simulink library "GEJenbacherJ620"  (Simulink 8.1)
settings: Solver=ode45  StartTime=0.0  StopTime=10.0  RelTol=1e-3
undefined symbols (not defined in the file): DiscIntNeverNeededParam, Ts
libraries: simulink x1
settings Model: Creator=ed12083  LastModifiedBy=ed12083

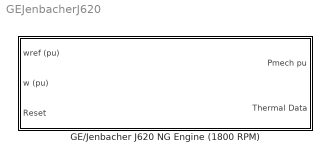
== system GEJenbacherJ620 ==
  GE/Jenbacher J620 NG Engine (1800 RPM) : Subsystem  mask{cd=.8, H=47133, keq=1.3962, Ma=.029, Meq=.0285, Mf=.019, P0=800000, Pm=37241, R=8.314, T0=300, Tm=325, thermalEfficiency=.45, V=0.031, Vd=0.125, volumeEfficiency=.9, P=3, I=3, UL=1.05, LL=0, UPL=1.05, LPL=0}
      mask prompts: cd "Discharge coefficient - cd"; H "NG heating value - H"; keq "Equivalent ratio of specific heats of air/fuel mixture - keq"; Ma "Molecular weight of air - Ma"; Meq "Equivalent molecular weight of air/fuel mixture - Meq"; Mf "Molecular weight of NG - Mf"; P0 "Throttle inlet air pressure - P0"; Pm "Intake manifold pressure - Pm"; R "Universal gas constant - R"; T0 "Throttle inlet charge temperature - T0"; Tm "Intake manifold temperature - Tm"; thermalEfficiency "Thermal efficiency - thermalEfficiency"; V "Manifold plus port passage volume - V"; Vd "Engine displacement - Vd"; volumeEfficiency "Volumetric efficiency - volumeEfficiency"; P "Proportional Gain - P"; I "Integral Gain - I"; UL "Upper Integrator Limit - UL"; LL "Lower Integrator Limit - LL"; UPL "Upper Power Limit - UPL"; LPL "Lower Power Limit - LPL"
      mask help: All units are MKS. Refer to "Modeling and Validation of a Lean Burn Natural Gas Engine", Gangopadhyay et. al., ASME 2001

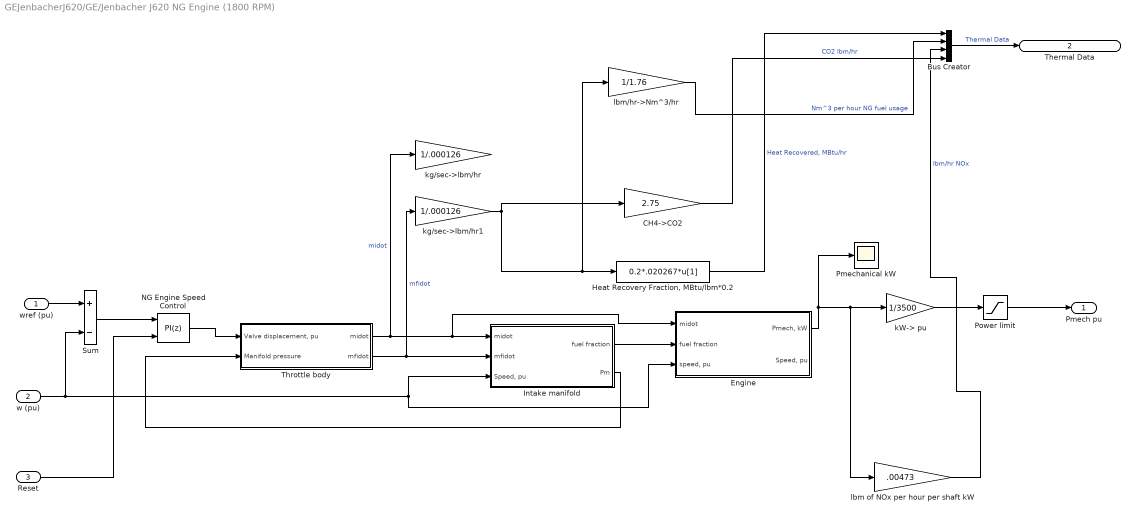
== system GEJenbacherJ620/GE/Jenbacher J620 NG Engine (1800 RPM) ==
  wref (pu) : Inport
  w (pu) : Inport  Port=2
  Reset : Inport  Port=3
  Bus Creator : BusCreator
  CH4->CO2 : Gain  Gain=2.75
  Engine : Subsystem
  "Heat Recovery Fraction, MBtu/lbm*0.2 " : Fcn  Expr=0.2*.020267*u[1]
  Intake manifold : Subsystem
  NG Engine Speed Control : simulink/Continuous/PID Controller  Controller=PI  TimeDomain=Discrete-time  SampleTime=Ts  IntegratorMethod=Forward Euler  FilterMethod=Forward Euler  Form=Parallel  P=P  I=I  D=0.5  N=10000  InitialConditionSource=internal  InitialConditionForIntegrator=0  InitialConditionForFilter=0  ExternalReset=rising  ZeroCross=off  LimitOutput=on  UpperSaturationLimit=UL  LowerSaturationLimit=LL  LinearizeAsGain=off  AntiWindupMode=back-calculation  Kb=1  TrackingMode=off  Kt=1  PParamMin=[]  PParamMax=[]  IParamMin=[]  IParamMax=[]  DParamMin=[]  DParamMax=[]  NParamMin=[]  NParamMax=[]  KbParamMin=[]  KbParamMax=[]  KtParamMin=[]  KtParamMax=[]  POutMin=[]  POutMax=[]  IOutMin=[]  IOutMax=[]  DOutMin=[]  DOutMax=[]  NOutMin=[]  NOutMax=[]  KbOutMin=[]  KbOutMax=[]  KtOutMin=[]  KtOutMax=[]  IntegratorOutMin=[]  IntegratorOutMax=[]  FilterOutMin=[]  FilterOutMax=[]  SumOutMin=[]  SumOutMax=[]  SumI1OutMin=[]  SumI1OutMax=[]  SumI2OutMin=[]  SumI2OutMax=[]  SumI3OutMin=[]  SumI3OutMax=[]  SumDOutMin=[]  SumDOutMax=[]  SaturationOutMin=[]  SaturationOutMax=[]  IntegratorContinuousStateAttributes=''  IntegratorStateMustResolveToSignalObject=off  IntegratorRTWStateStorageClass=Auto  FilterContinuousStateAttributes=''  FilterStateMustResolveToSignalObject=off  FilterRTWStateStorageClass=Auto
  Pmechanical kW : Scope
      settings: TimeRange=10  YMin=0  YMax=4500  SaveName=ScopeData9
  Power limit : Saturate  UpperLimit=UPL  LowerLimit=LPL
  Sum : Sum  Inputs=+-  SaturateOnIntegerOverflow=on  InputSameDT=on  OutDataTypeStr=Inherit: Same as first input
  Throttle body : Subsystem
  kW-> pu : Gain  Gain=1/3500
  kg/sec->lbm/hr : Gain  Gain=1/.000126
  kg/sec->lbm/hr1 : Gain  Gain=1/.000126
  lbm of NOx per hour per shaft kW : Gain  Gain=.00473
  lbm/hr->Nm^3/hr : Gain  Gain=1/1.76
  Pmech pu : Outport
  Thermal Data : Outport  Port=2
  wires:
  CH4->CO2/1 -> Bus Creator/4  "CO2 lbm/hr"
  Bus Creator/1 -> Thermal Data/1  "Thermal Data"
  w (pu)/1 -> Sum/2, Intake manifold/3("Speed, pu"), Engine/3("speed, pu")
  Intake manifold/1(fuel fraction) -> Engine/2(fuel fraction)
  Intake manifold/2(Pm) -> Throttle body/2("Manifold pressure ")
  Throttle body/1(midot) -> kg/sec->lbm/hr/1, Engine/1(midot), Intake manifold/1(midot)  "midot"
  Engine/1("Pmech, kW") -> Pmechanical kW/1, lbm of NOx per hour per shaft kW/1, kW-> pu/1
  kg/sec->lbm/hr1/1 -> CH4->CO2/1, lbm/hr->Nm^3/hr/1, "Heat Recovery Fraction, MBtu/lbm*0.2 "/1
  Throttle body/2(mfidot) -> kg/sec->lbm/hr1/1, Intake manifold/2(mfidot)  "mfidot"
  "Heat Recovery Fraction, MBtu/lbm*0.2 "/1 -> Bus Creator/1  "Heat Recovered, MBtu/hr"
  lbm/hr->Nm^3/hr/1 -> Bus Creator/2  "Nm^3 per hour NG fuel usage"
  lbm of NOx per hour per shaft kW/1 -> Bus Creator/3  "lbm/hr NOx"
  kW-> pu/1 -> Power limit/1
  Power limit/1 -> Pmech pu/1
  wref (pu)/1 -> Sum/1
  NG Engine Speed Control/1 -> Throttle body/1("Valve displacement, pu")
  Sum/1 -> NG Engine Speed Control/1
  Reset/1 -> NG Engine Speed Control/2

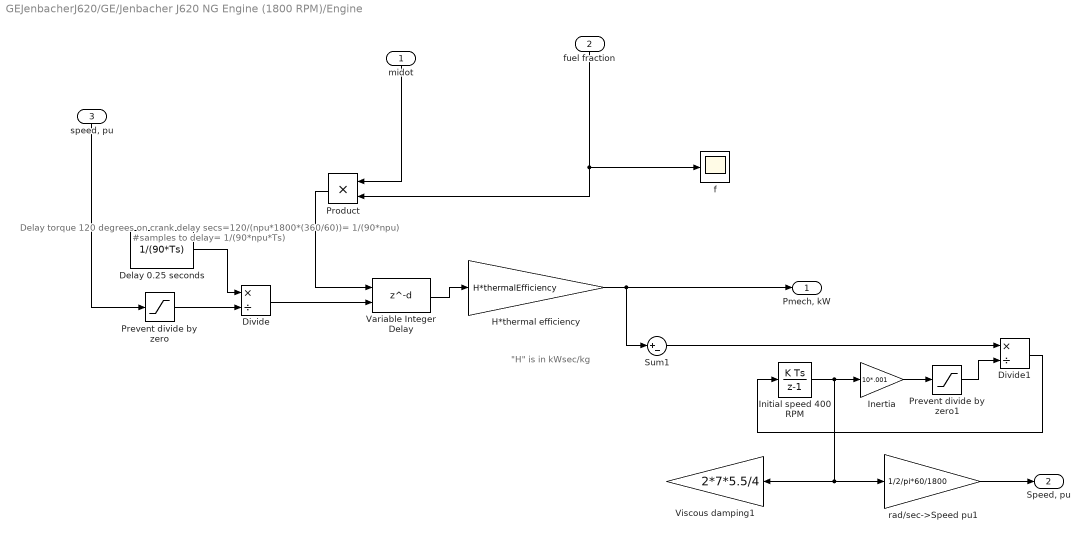
== system GEJenbacherJ620/GE/Jenbacher J620 NG Engine (1800 RPM)/Engine ==
  note: "H" is in kWsec/kg
  note: Delay torque 120 degrees on crank
      | delay secs=120/(npu*1800*(360/60))= 1/(90*npu)
      | #samples to delay= 1/(90*npu*Ts)
  midot : Inport
  fuel fraction : Inport  Port=2
  "speed, pu" : Inport  Port=3
  Delay 0.25 seconds : Constant  Value=1/(90*Ts)
  Divide : Product  Inputs=*/
  Divide1 : Product  Inputs=*/
  H*thermal efficiency : Gain  Gain=H*thermalEfficiency
  Inertia : Gain  Gain=10*.001
  Initial speed 400 RPM : DiscreteIntegrator  gainval=1  InitialCondition=10/60*2*pi  SampleTime=Ts  LimitOutput=on  LowerSaturationLimit=0  ICPrevOutput=DiscIntNeverNeededParam  ICPrevScaledInput=DiscIntNeverNeededParam
  Prevent divide by zero : Saturate  UpperLimit=inf  LowerLimit=.001
  Prevent divide by zero1 : Saturate  UpperLimit=inf  LowerLimit=.001
  Product : Product
  Sum1 : Sum  Inputs=|+-
  Variable Integer Delay : Delay  DelayLengthSource=Input port  SampleTime=Ts
      settings: InputPortMap=u0,p1
  Viscous damping1 : Gain  Gain=2*7*5.5/4
  f : Scope
      settings: YMin=0.0452381  YMax=0.05  SaveName=ScopeData3
  rad/sec->Speed pu1 : Gain  Gain=1/2/pi*60/1800
  "Pmech, kW" : Outport
  "Speed, pu " : Outport  Port=2
  wires:
  fuel fraction/1 -> f/1, Product/2
  Product/1 -> Variable Integer Delay/1
  Variable Integer Delay/1 -> H*thermal efficiency/1
  Prevent divide by zero/1 -> Divide/2
  midot/1 -> Product/1
  Delay 0.25 seconds/1 -> Divide/1
  Divide/1 -> Variable Integer Delay/2
  Initial speed 400 RPM/1 -> Viscous damping1/1, rad/sec->Speed pu1/1, Inertia/1
  Inertia/1 -> Prevent divide by zero1/1
  Divide1/1 -> Initial speed 400 RPM/1
  rad/sec->Speed pu1/1 -> "Speed, pu "/1
  Sum1/1 -> Divide1/1
  "speed, pu"/1 -> Prevent divide by zero/1
  Prevent divide by zero1/1 -> Divide1/2
  H*thermal efficiency/1 -> "Pmech, kW"/1, Sum1/1

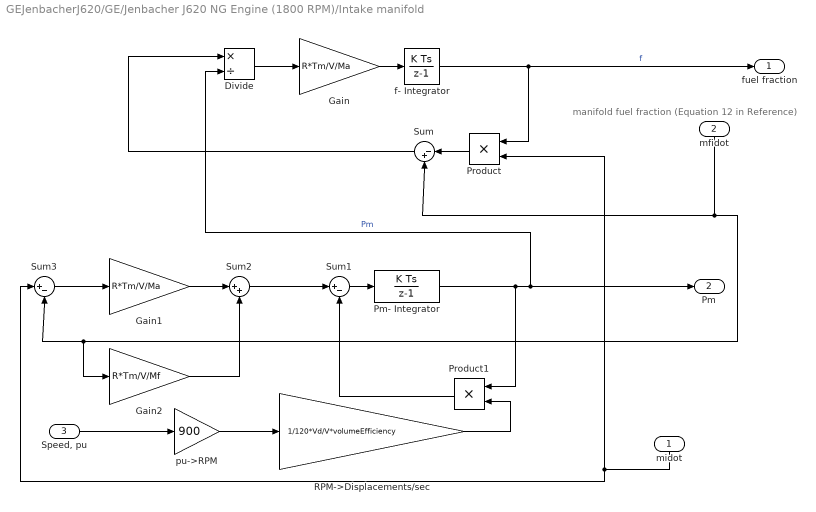
== system GEJenbacherJ620/GE/Jenbacher J620 NG Engine (1800 RPM)/Intake manifold ==
  note: manifold fuel fraction
      | (Equation 12 in Reference)
  midot : Inport
  mfidot : Inport  Port=2
  "Speed, pu" : Inport  Port=3
  Divide : Product  Inputs=*/
  Gain : Gain  Gain=R*Tm/V/Ma
  Gain1 : Gain  Gain=R*Tm/V/Ma
  Gain2 : Gain  Gain=R*Tm/V/Mf
  Pm- Integrator : DiscreteIntegrator  InitialCondition=.8/.000145  SampleTime=Ts  LimitOutput=on  UpperSaturationLimit=400000  LowerSaturationLimit=0  ICPrevOutput=DiscIntNeverNeededParam  ICPrevScaledInput=DiscIntNeverNeededParam
  Product : Product
  Product1 : Product
  RPM->Displacements/sec : Gain  Gain=1/120*Vd/V*volumeEfficiency
  Sum : Sum  Inputs=|-+
  Sum1 : Sum  Inputs=|+-
  Sum2 : Sum  Inputs=|++
  Sum3 : Sum  Inputs=|+-
  "f- Integrator " : DiscreteIntegrator  InitialCondition=1/21  SampleTime=Ts  ICPrevOutput=DiscIntNeverNeededParam  ICPrevScaledInput=DiscIntNeverNeededParam
  pu->RPM : Gain  Gain=900
  fuel fraction : Outport
  Pm : Outport  Port=2
  wires:
  Gain/1 -> "f- Integrator "/1
  Divide/1 -> Gain/1
  "f- Integrator "/1 -> fuel fraction/1, Product/1  "f"
  Product/1 -> Sum/1
  Sum/1 -> Divide/1
  Sum1/1 -> Pm- Integrator/1
  Pm- Integrator/1 -> Divide/2, Pm/1, Product1/1  "Pm"
  "Speed, pu"/1 -> pu->RPM/1
  pu->RPM/1 -> RPM->Displacements/sec/1
  midot/1 -> Product/2, Sum3/1
  Product1/1 -> Sum1/2
  RPM->Displacements/sec/1 -> Product1/2
  mfidot/1 -> Sum/2, Gain2/1, Sum3/2
  Gain1/1 -> Sum2/1
  Sum2/1 -> Sum1/1
  Sum3/1 -> Gain1/1
  Gain2/1 -> Sum2/2

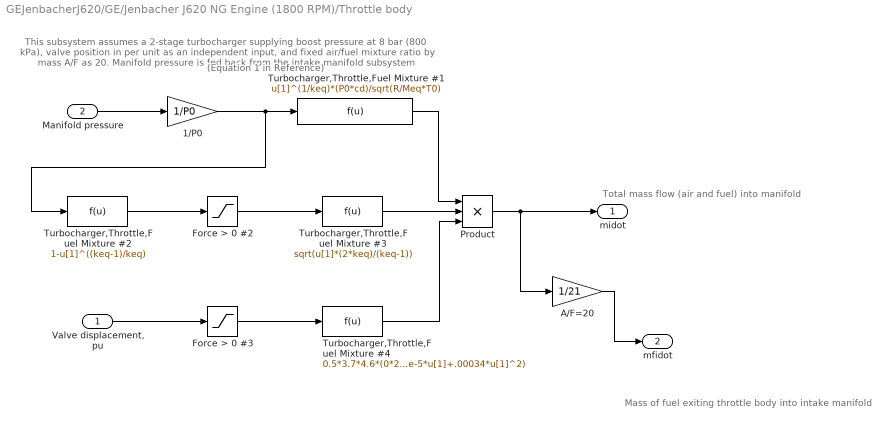
== system GEJenbacherJ620/GE/Jenbacher J620 NG Engine (1800 RPM)/Throttle body ==
  note: Mass of fuel exiting throttle body into intake manifold
  note: This subsystem assumes a 2-stage turbocharger supplying boost pressure at 8 bar (800 kPa),
      | valve position in per unit as an independent input, and fixed air/fuel mixture ratio by mass A/F as 20.
      | Manifold pressure is fed back from the intake manifold subsystem
  note: Total mass flow (air and fuel) into manifold
  note: (Equation 1 in Reference)
  "Valve displacement, pu" : Inport
  "Manifold pressure " : Inport  Port=2
  1/P0 : Gain  Gain=1/P0
  A/F=20 : Gain  Gain=1/21
  Force > 0 #2 : Saturate  UpperLimit=inf  LowerLimit=0
  Force > 0 #3 : Saturate  UpperLimit=1  LowerLimit=0
  Product : Product  Inputs=3
  Turbocharger,Throttle,Fuel Mixture #1 : Fcn  Expr=u[1]^(1/keq)*(P0*cd)/sqrt(R/Meq*T0)
  Turbocharger,Throttle,Fuel Mixture #2 : Fcn  Expr=1-u[1]^((keq-1)/keq)
  Turbocharger,Throttle,Fuel Mixture #3 : Fcn  Expr=sqrt(u[1]*(2*keq)/(keq-1))
  Turbocharger,Throttle,Fuel Mixture #4 : Fcn  Expr=0.5*3.7*4.6*(0*2.9e-5+3.2e-5*u[1]+.00034*u[1]^2)
  midot : Outport
  mfidot : Outport  Port=2
  wires:
  "Manifold pressure "/1 -> 1/P0/1
  A/F=20/1 -> mfidot/1
  Turbocharger,Throttle,Fuel Mixture #2/1 -> Force > 0 #2/1
  Force > 0 #2/1 -> Turbocharger,Throttle,Fuel Mixture #3/1
  "Valve displacement, pu"/1 -> Force > 0 #3/1
  Turbocharger,Throttle,Fuel Mixture #1/1 -> Product/1
  Turbocharger,Throttle,Fuel Mixture #3/1 -> Product/2
  Turbocharger,Throttle,Fuel Mixture #4/1 -> Product/3
  Product/1 -> A/F=20/1, midot/1
  Force > 0 #3/1 -> Turbocharger,Throttle,Fuel Mixture #4/1
  1/P0/1 -> Turbocharger,Throttle,Fuel Mixture #2/1, Turbocharger,Throttle,Fuel Mixture #1/1
